simulink model "simulinkCS"  (Simulink 7.4)
settings: Solver=ode45  StartTime=0.0  StopTime=10.0  RelTol=1e-3
(part 1 of 2)
settings Model: Creator=Kubik  LastModifiedBy=Kubik

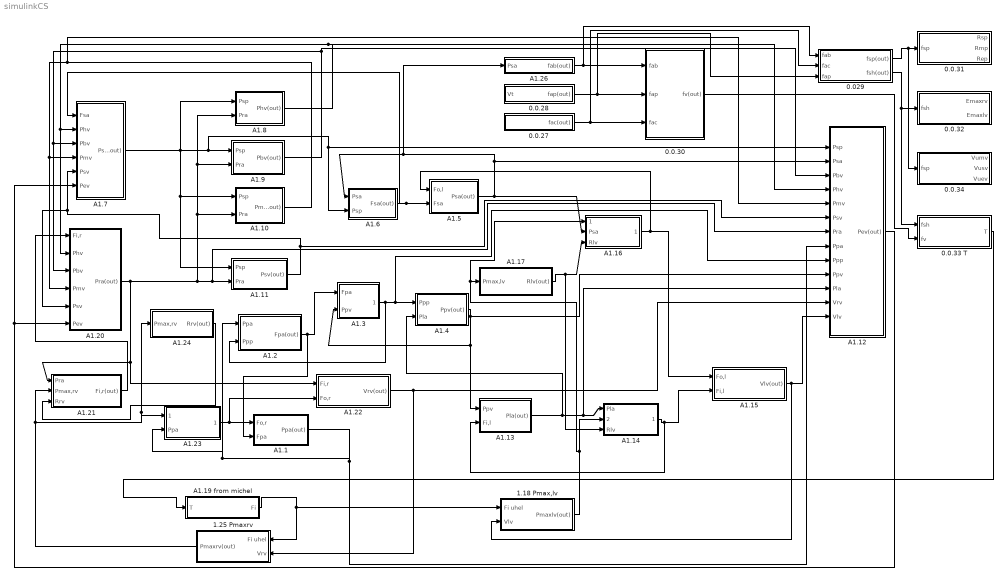
== system simulinkCS ==
  0.0.27 : Subsystem
  0.0.28 : Subsystem
  0.0.30 : Subsystem
  0.0.31 : Subsystem
  0.0.32 : Subsystem
  0.0.33 T : Subsystem
  0.0.34 : Subsystem
  0.029 : Subsystem
  1.18 Pmax,lv : Subsystem
  1.25 Pmaxrv : Subsystem
  A1.1 : Subsystem
  A1.10 : Subsystem
  A1.11 : Subsystem
  A1.12 : Subsystem
  A1.13 : Subsystem
  A1.14 : Subsystem
  A1.15 : Subsystem
  A1.16 : Subsystem
  A1.17 : Subsystem
  A1.19 from michel : Subsystem
  A1.2 : Subsystem
  A1.20 : Subsystem
  A1.21 : Subsystem
  A1.22 : Subsystem
  A1.23 : Subsystem
  A1.24 : Subsystem
  A1.26 : Subsystem
  A1.3 : Subsystem
  A1.4 : Subsystem
  A1.5 : Subsystem
  A1.6 : Subsystem
  A1.7 : Subsystem
  A1.8 : Subsystem
  A1.9 : Subsystem
  wires:
  A1.14/1(Fi,l(out)) -> A1.15/2(Fi,l), A1.13/2(Fi,l)
  A1.16/1(Fo,l(out)) -> A1.15/1(Fo,l), A1.5/1(Fo,l)
  A1.17/1(Rlv(out)) -> A1.16/3(Rlv), A1.14/3(Rlv)
  A1.5/1(Psa(out)) -> A1.16/2(Psa), A1.6/1(Psa), A1.26/1(Psa), A1.12/2(Psa)
  A1.13/1(Pla(out)) -> A1.4/2(Pla), A1.14/1(Pla), A1.12/11(Pla)
  A1.20/1(Pra(out)) -> A1.10/2(Pra), A1.9/2(Pra), A1.8/2(Pra), A1.11/2(Pra), A1.12/7(Pra), A1.21/1(Pra), A1.22/1(Fi,r)
  A1.7/1(Psp(out)) -> A1.8/1(Psp), A1.10/1(Psp), A1.11/1(Psp), A1.9/1(Psp), A1.6/2(Psp), A1.12/1(Psp)
  A1.15/1(Vlv(out)) -> A1.12/13(Vlv), 1.18 Pmax,lv/2(Vlv)
  A1.6/1(Fsa(out)) -> A1.5/2(Fsa), A1.7/1(Fsa)
  A1.21/1(Fi,r(out)) -> A1.20/1(Fi,r)
  A1.23/1(Fo,r(out)) -> A1.1/1(Fo,r), A1.22/2(Fo,r)
  A1.1/1(Ppa(out)) -> A1.23/2(Ppa), A1.2/1(Ppa), A1.12/8(Ppa)
  A1.22/1(Vrv(out)) -> A1.12/12(Vrv), 1.25 Pmaxrv/2(Vrv)
  A1.4/1(Ppv(out)) -> A1.13/1(Ppv), A1.3/2(Ppv), A1.12/10(Ppv)
  A1.3/1(Ppp(out)) -> A1.2/2(Ppp), A1.4/1(Ppp), A1.12/9(Ppp)
  A1.26/1(fab(out)) -> 0.0.30/1(fab), 0.029/1(fab)
  A1.2/1(Fpa(out)) -> A1.3/1(Fpa), A1.1/2(Fpa)
  A1.11/1(Psv(out)) -> A1.7/5(Psv), A1.20/5(Psv), A1.12/6(Psv)
  A1.10/1(Pmv(out)) -> A1.7/4(Pmv), A1.20/4(Pmv), A1.12/5(Pmv)
  A1.9/1(Pbv(out)) -> A1.7/3(Pbv), A1.20/3(Pbv), A1.12/3(Pbv)
  A1.8/1(Phv(out)) -> A1.7/2(Phv), A1.20/2(Phv), A1.12/4(Phv)
  0.0.27/1(fac(out)) -> 0.0.30/3(fac), 0.029/2(fac)
  0.0.28/1(fap(out)) -> 0.0.30/2(fap), 0.029/3(fap)
  A1.12/1(Pev(out)) -> A1.20/6(Pev), A1.7/6(Pev)
  A1.24/1(Rrv(out)) -> A1.21/3(Rrv)
  A1.19 from michel/1(Fi) -> 1.25 Pmaxrv/1(Fi uhel), 1.18 Pmax,lv/1(Fi uhel)
  1.25 Pmaxrv/1(Pmaxrv(out)) -> A1.21/2(Pmax,rv), A1.24/1(Pmax,rv), A1.23/1(Pmax,rv)
  1.18 Pmax,lv/1(Pmaxlv(out)) -> A1.14/2(Pmax,lv), A1.17/1(Pmax,lv), A1.16/1(Pmax,lv)
  0.029/1(fsp(out)) -> 0.0.31/1(fsp), 0.0.34/1(fsp)
  0.029/2(fsh(out)) -> 0.0.32/1(fsh), 0.0.33 T/1(fsh)
  0.0.30/1(fv(out)) -> 0.0.33 T/2(fv)
  0.0.33 T/1(T) -> A1.19 from michel/1(T)

== system simulinkCS/0.0.27 ==
  1 : Constant  OutDataType=fixdt(1, 16)  OutScaling=2^0
  Add : Sum  OutDataType=fixdt(1, 16)  OutScaling=2^-10
  Add1 : Sum  Inputs=+-  OutDataType=fixdt(1, 16)  OutScaling=2^-10
  Add2 : Sum  OutDataType=fixdt(1, 16)  OutScaling=2^-10
  Add4 : Sum  Inputs=-+  OutDataType=fixdt(1, 16)  OutScaling=2^-10
  Divide : Product  Inputs=*/  OutDataType=fixdt(1, 16)  OutScaling=2^-10
  Divide1 : Product  Inputs=*/  OutDataType=fixdt(1, 16)  OutScaling=2^-10
  Divide2 : Product  Inputs=*/  OutDataType=fixdt(1, 16)  OutScaling=2^-10
  Integrator1 : Integrator
  Math Function : Math  OutDataType=fixdt(1, 16)  OutScaling=2^0  SaturateOnIntegerOverflow=on
  Pas,O2 : Constant  Value=35  OutMin=30  OutMax=110  OutDataType=fixdt(1, 16)  OutScaling=2^0
  Pas,O2n : Constant  Value=45  OutDataType=fixdt(1, 16)  OutScaling=2^0
  Product : Product  OutDataType=fixdt(1, 16)  OutScaling=2^0  RndMeth=Zero
  fac,max : Constant  Value=2.52  OutDataType=fixdt(1, 16)  OutScaling=2^0
  fac,min : Constant  Value=47.78  OutDataType=fixdt(1, 16)  OutScaling=2^0
  kac : Constant  Value=29.27  OutDataType=fixdt(1, 16)  OutScaling=2^0
  tau-c : Constant  OutDataType=fixdt(1, 16)  OutScaling=2^0
  fac(out) : Outport  OutDataType=fixdt(1, 16)  OutScaling=2^0
  wires:
  Integrator1/1 -> fac(out)/1, Add4/1
  Add4/1 -> Divide2/1
  Divide2/1 -> Integrator1/1
  tau-c/1 -> Divide2/2
  fac,min/1 -> Product/1
  Math Function/1 -> Product/2, Add2/1
  Add/1 -> Divide/1
  Product/1 -> Add/2
  fac,max/1 -> Add/1
  1/1 -> Add2/2
  Add2/1 -> Divide/2
  Divide/1 -> Add4/2
  Add1/1 -> Divide1/1
  kac/1 -> Divide1/2
  Divide1/1 -> Math Function/1
  Pas,O2n/1 -> Add1/2
  Pas,O2/1 -> Add1/1

== system simulinkCS/0.0.28 ==
  Vt : Inport  OutDataType=fixdt(1, 16)  OutScaling=2^0
  Add4 : Sum  Inputs=-+  OutDataType=fixdt(1, 16)  OutScaling=2^-10
  Divide2 : Product  Inputs=*/  OutDataType=fixdt(1, 16)  OutScaling=2^-10
  Gap : Constant  Value=1000/23291  OutDataType=fixdt(1, 16)  OutScaling=2^0
  Integrator1 : Integrator
  Product : Product  OutDataType=fixdt(1, 16)  OutScaling=2^0  RndMeth=Zero
  tau-c : Constant  OutDataType=fixdt(1, 16)  OutScaling=2^0
  fap(out) : Outport  OutDataType=fixdt(1, 16)  OutScaling=2^0
  wires:
  Integrator1/1 -> fap(out)/1, Add4/1
  Add4/1 -> Divide2/1
  Divide2/1 -> Integrator1/1
  tau-c/1 -> Divide2/2
  Gap/1 -> Product/1
  Product/1 -> Add4/2
  Vt/1 -> Product/2

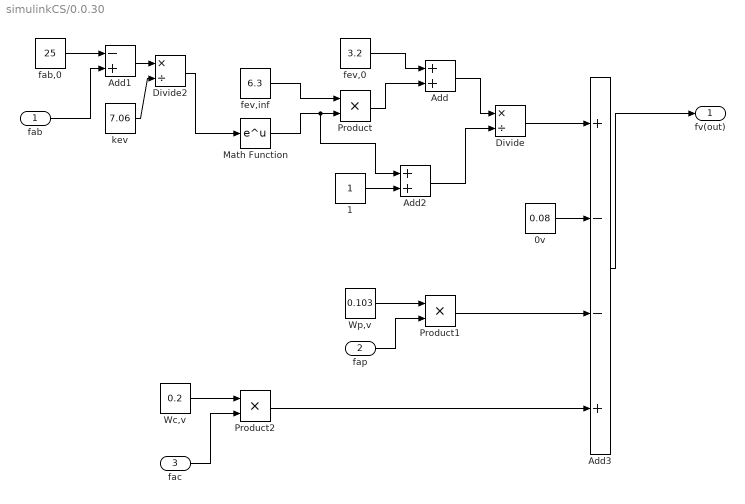
== system simulinkCS/0.0.30 ==
  fab : Inport  OutDataType=fixdt(1, 16)  OutScaling=2^0
  fap : Inport  Port=2  OutDataType=fixdt(1, 16)  OutScaling=2^0
  fac : Inport  Port=3  OutDataType=fixdt(1, 16)  OutScaling=2^0
  0v : Constant  Value=0.08  OutDataType=fixdt(1, 16)  OutScaling=2^0
  1 : Constant  OutDataType=fixdt(1, 16)  OutScaling=2^0
  Add : Sum  OutDataType=fixdt(1, 16)  OutScaling=2^-10
  Add1 : Sum  Inputs=-+  OutDataType=fixdt(1, 16)  OutScaling=2^-10
  Add2 : Sum  OutDataType=fixdt(1, 16)  OutScaling=2^-10
  Add3 : Sum  Inputs=+--+  OutDataType=fixdt(1, 16)  OutScaling=2^-10
  Divide : Product  Inputs=*/  OutDataType=fixdt(1, 16)  OutScaling=2^-10
  Divide2 : Product  Inputs=*/  OutDataType=fixdt(1, 16)  OutScaling=2^-10
  Math Function : Math  OutDataType=fixdt(1, 16)  OutScaling=2^0  SaturateOnIntegerOverflow=on
  Product : Product  OutDataType=fixdt(1, 16)  OutScaling=2^0  RndMeth=Zero
  Product1 : Product  OutDataType=fixdt(1, 16)  OutScaling=2^0  RndMeth=Zero
  Product2 : Product  OutDataType=fixdt(1, 16)  OutScaling=2^0  RndMeth=Zero
  Wc,v : Constant  Value=0.2  OutDataType=fixdt(1, 16)  OutScaling=2^0
  Wp,v : Constant  Value=0.103  OutDataType=fixdt(1, 16)  OutScaling=2^0
  fab,0 : Constant  Value=25  OutDataType=fixdt(1, 16)  OutScaling=2^0
  fev,0 : Constant  Value=3.2  OutDataType=fixdt(1, 16)  OutScaling=2^0
  fev,inf : Constant  Value=6.3  OutDataType=fixdt(1, 16)  OutScaling=2^0
  kev : Constant  Value=7.06  OutDataType=fixdt(1, 16)  OutScaling=2^0
  fv(out) : Outport  OutDataType=fixdt(1, 16)  OutScaling=2^0
  wires:
  fev,inf/1 -> Product/1
  Math Function/1 -> Product/2, Add2/1
  Add/1 -> Divide/1
  Product/1 -> Add/2
  fev,0/1 -> Add/1
  Add1/1 -> Divide2/1
  Divide2/1 -> Math Function/1
  kev/1 -> Divide2/2
  fab,0/1 -> Add1/1
  1/1 -> Add2/2
  Add2/1 -> Divide/2
  fab/1 -> Add1/2
  Divide/1 -> Add3/1
  Add3/1 -> fv(out)/1
  0v/1 -> Add3/2
  Wp,v/1 -> Product1/1
  Wc,v/1 -> Product2/1
  Product1/1 -> Add3/3
  Product2/1 -> Add3/4
  fap/1 -> Product1/2
  fac/1 -> Product2/2

== system simulinkCS/0.0.31 ==
  fsp : Inport  OutDataType=sfix(16)  OutScaling=2^0
  Rep sub : Subsystem
  Rmp sub : Subsystem
  Rsp sub : Subsystem
  Rsp : Outport  OutDataType=sfix(16)  OutScaling=2^0
  Rmp : Outport  Port=2  OutDataType=sfix(16)  OutScaling=2^0
  Rep : Outport  Port=3  OutDataType=sfix(16)  OutScaling=2^0
  wires:
  fsp/1 -> Rsp sub/1(fsp), Rmp sub/1(fsp), Rep sub/1(fsp)
  Rsp sub/1(Rsp) -> Rsp/1
  Rmp sub/1(Rmp) -> Rmp/1
  Rep sub/1(Rep) -> Rep/1

== system simulinkCS/0.0.32 ==
  fsh : Inport  OutDataType=sfix(16)  OutScaling=2^0
  Rmp sub : Subsystem
  Rsp sub : Subsystem
  Emaxrv : Outport  OutDataType=sfix(16)  OutScaling=2^0
  Emaxlv : Outport  Port=2  OutDataType=sfix(16)  OutScaling=2^0
  wires:
  fsh/1 -> Rsp sub/1(fsh), Rmp sub/1(fsh)
  Rsp sub/1(Emaxrv) -> Emaxrv/1
  Rmp sub/1(Emaxlv) -> Emaxlv/1

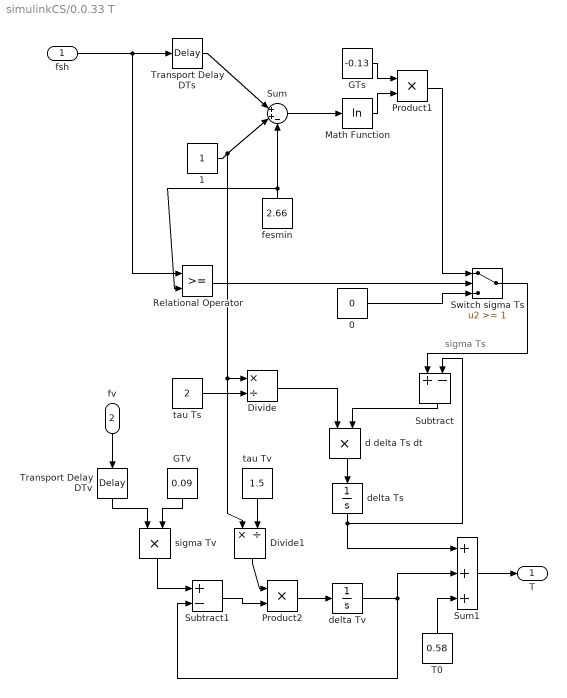
== system simulinkCS/0.0.33 T ==
  note: sigma Ts
  fsh : Inport  OutDataType=sfix(16)  OutScaling=2^0
  fv : Inport  Port=2  OutDataType=sfix(16)  OutScaling=2^0
  0 : Constant  Value=0  OutDataType=sfix(16)  OutScaling=2^0
  1 : Constant  OutDataType=sfix(16)  OutScaling=2^0
  Divide : Product  Inputs=*/  OutDataType=sfix(16)  OutScaling=2^-10
  Divide1 : Product  Inputs=*/  OutDataType=sfix(16)  OutScaling=2^-10
  GTs : Constant  Value=-0.13  OutDataType=sfix(16)  OutScaling=2^0
  GTv : Constant  Value=0.09  OutDataType=sfix(16)  OutScaling=2^0
  Math Function : Math  Operator=log  OutDataType=sfix(16)  OutScaling=2^0  SaturateOnIntegerOverflow=on
  Product1 : Product  OutDataType=sfix(16)  OutScaling=2^0  RndMeth=Zero
  Product2 : Product  OutDataType=sfix(16)  OutScaling=2^0  RndMeth=Zero
  Relational Operator : RelationalOperator  LogicOutDataTypeMode=boolean  OutDataTypeStr=boolean
  Subtract : Sum  Inputs=+-  OutDataType=sfix(16)  OutScaling=2^-10
  Subtract1 : Sum  Inputs=+-  OutDataType=sfix(16)  OutScaling=2^-10
  Sum : Sum  Inputs=|++-  OutDataType=sfix(16)  OutScaling=2^0
  Sum1 : Sum  Inputs=+++  OutDataType=sfix(16)  OutScaling=2^0
  Switch sigma Ts : Switch  Threshold=1
  T0 : Constant  Value=0.58  OutDataType=sfix(16)  OutScaling=2^0
  Transport Delay DTs : TransportDelay  DelayTime=2
  Transport Delay DTv : TransportDelay  DelayTime=0.2
  "d delta Ts dt  " : Product  OutDataType=sfix(16)  OutScaling=2^0  RndMeth=Zero
  delta Ts : Integrator
  delta Tv : Integrator
  fesmin : Constant  Value=2.66  OutDataType=sfix(16)  OutScaling=2^0
  sigma Tv : Product  OutDataType=sfix(16)  OutScaling=2^0  RndMeth=Zero
  tau Ts : Constant  Value=2  OutDataType=sfix(16)  OutScaling=2^0
  tau Tv : Constant  Value=1.5  OutDataType=sfix(16)  OutScaling=2^0
  T : Outport  OutDataType=sfix(16)  OutScaling=2^0
  wires:
  fsh/1 -> Transport Delay DTs/1, Relational Operator/1
  GTs/1 -> Product1/1
  1/1 -> Sum/2, Divide/1, Divide1/1
  fesmin/1 -> Sum/3, Relational Operator/2
  Transport Delay DTs/1 -> Sum/1
  Sum/1 -> Math Function/1
  Math Function/1 -> Product1/2
  Product1/1 -> Switch sigma Ts/1
  Relational Operator/1 -> Switch sigma Ts/2
  0/1 -> Switch sigma Ts/3
  Switch sigma Ts/1 -> Subtract/1
  tau Ts/1 -> Divide/2
  delta Ts/1 -> Subtract/2, Sum1/1
  Subtract/1 -> "d delta Ts dt  "/2
  Divide/1 -> "d delta Ts dt  "/1
  "d delta Ts dt  "/1 -> delta Ts/1
  fv/1 -> Transport Delay DTv/1
  Transport Delay DTv/1 -> sigma Tv/1
  GTv/1 -> sigma Tv/2
  tau Tv/1 -> Divide1/2
  sigma Tv/1 -> Subtract1/1
  delta Tv/1 -> Subtract1/2, Sum1/2
  Product2/1 -> delta Tv/1
  Subtract1/1 -> Product2/2
  Divide1/1 -> Product2/1
  T0/1 -> Sum1/3
  Sum1/1 -> T/1

== system simulinkCS/0.0.34 ==
  fsp : Inport  OutDataType=sfix(16)  OutScaling=2^0
  Vumv sub : Subsystem
  Vumv sub1 : Subsystem
  Vumv sub2 : Subsystem
  Vumv : Outport  OutDataType=sfix(16)  OutScaling=2^0
  Vusv : Outport  Port=2  OutDataType=sfix(16)  OutScaling=2^0
  Vuev : Outport  Port=3  OutDataType=sfix(16)  OutScaling=2^0
  wires:
  fsp/1 -> Vumv sub/1(fsp), Vumv sub1/1(fsp), Vumv sub2/1(fsp)
  Vumv sub/1(Vumv) -> Vumv/1
  Vumv sub1/1(Vusv) -> Vusv/1
  Vumv sub2/1(Vuev) -> Vuev/1

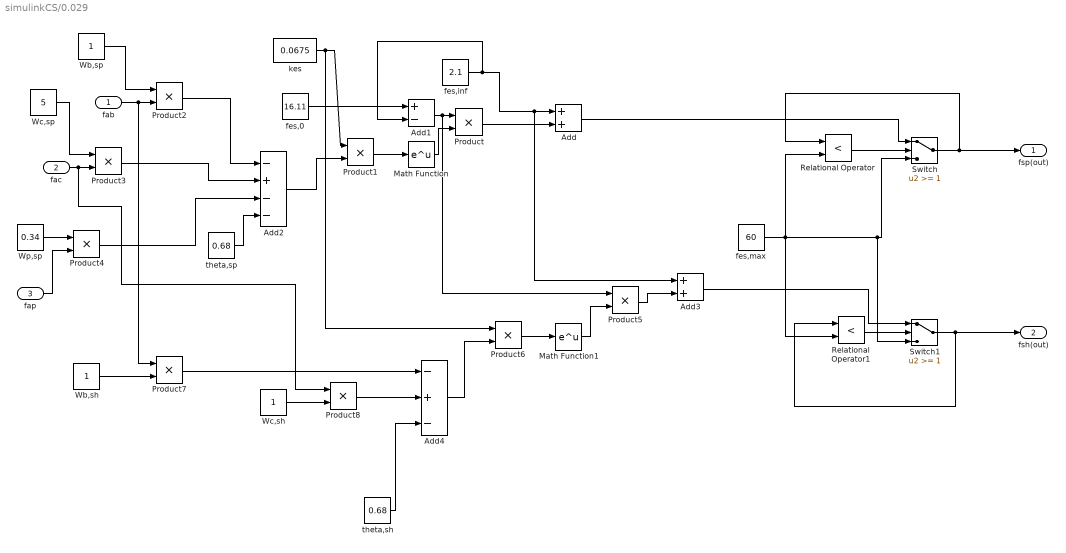
== system simulinkCS/0.029 ==
  fab : Inport  OutDataType=fixdt(1, 16)  OutScaling=2^0
  fac : Inport  Port=2  OutDataType=fixdt(1, 16)  OutScaling=2^0
  fap : Inport  Port=3  OutDataType=fixdt(1, 16)  OutScaling=2^0
  Add : Sum  OutDataType=fixdt(1, 16)  OutScaling=2^-10
  Add1 : Sum  Inputs=+-  OutDataType=fixdt(1, 16)  OutScaling=2^-10
  Add2 : Sum  Inputs=-+--  OutDataType=fixdt(1, 16)  OutScaling=2^-10
  Add3 : Sum  OutDataType=fixdt(1, 16)  OutScaling=2^-10
  Add4 : Sum  Inputs=-+-  OutDataType=fixdt(1, 16)  OutScaling=2^-10
  Math Function : Math  OutDataType=fixdt(1, 16)  OutScaling=2^0  SaturateOnIntegerOverflow=on
  Math Function1 : Math  OutDataType=fixdt(1, 16)  OutScaling=2^0  SaturateOnIntegerOverflow=on
  Product{,1..8} (9 alike) : Product  OutDataType=fixdt(1, 16)  OutScaling=2^0  RndMeth=Zero
  Relational Operator : RelationalOperator  Operator=<  LogicOutDataTypeMode=boolean  LogicDataType=fixdt(0, 8)  OutDataTypeStr=boolean
  Relational Operator1 : RelationalOperator  Operator=<  LogicOutDataTypeMode=boolean  LogicDataType=fixdt(0, 8)  OutDataTypeStr=boolean
  Switch : Switch  Threshold=1  OutDataType=fixdt(1, 16)  OutScaling=2^0
  Switch1 : Switch  Threshold=1  OutDataType=fixdt(1, 16)  OutScaling=2^0
  Wb,sh : Constant  OutDataType=fixdt(1, 16)  OutScaling=2^0
  Wb,sp : Constant  OutDataType=fixdt(1, 16)  OutScaling=2^0
  Wc,sh : Constant  OutDataType=fixdt(1, 16)  OutScaling=2^0
  Wc,sp : Constant  Value=5  OutDataType=fixdt(1, 16)  OutScaling=2^0
  Wp,sp : Constant  Value=0.34  OutDataType=fixdt(1, 16)  OutScaling=2^0
  fes,0 : Constant  Value=16.11  OutDataType=fixdt(1, 16)  OutScaling=2^0
  fes,inf : Constant  Value=2.1  OutDataType=fixdt(1, 16)  OutScaling=2^0
  fes,max : Constant  Value=60  OutDataType=fixdt(1, 16)  OutScaling=2^0
  kes : Constant  Value=0.0675  OutDataType=fixdt(1, 16)  OutScaling=2^0
  theta,sh : Constant  Value=0.68  OutDataType=fixdt(1, 16)  OutScaling=2^0
  theta,sp : Constant  Value=0.68  OutDataType=fixdt(1, 16)  OutScaling=2^0
  fsp(out) : Outport  OutDataType=fixdt(1, 16)  OutScaling=2^0
  fsh(out) : Outport  Port=2  OutDataType=fixdt(1, 16)  OutScaling=2^0
  wires:
  Switch/1 -> fsp(out)/1, Relational Operator/1
  Switch1/1 -> fsh(out)/1, Relational Operator1/1
  fes,max/1 -> Switch1/3, Switch/3, Relational Operator/2, Relational Operator1/2
  Relational Operator1/1 -> Switch1/2
  Relational Operator/1 -> Switch/2
  Add1/1 -> Product/1, Product5/1
  Product/1 -> Add/2
  fes,inf/1 -> Add1/2, Add/1, Add3/1
  Math Function/1 -> Product/2
  Add/1 -> Switch/1
  fes,0/1 -> Add1/1
  Product1/1 -> Math Function/1
  Add2/1 -> Product1/2
  kes/1 -> Product1/1, Product6/1
  Product2/1 -> Add2/1
  fab/1 -> Product2/2, Product7/1
  Product3/1 -> Add2/2
  fac/1 -> Product3/2, Product8/1
  Product4/1 -> Add2/3
  theta,sp/1 -> Add2/4
  Wp,sp/1 -> Product4/1
  Wb,sp/1 -> Product2/1
  Add3/1 -> Switch1/1
  Product5/1 -> Add3/2
  Math Function1/1 -> Product5/2
  Product6/1 -> Math Function1/1
  Add4/1 -> Product6/2
  theta,sh/1 -> Add4/3
  Product7/1 -> Add4/1
  Wb,sh/1 -> Product7/2
  Wc,sp/1 -> Product3/1
  fap/1 -> Product4/2
  Product8/1 -> Add4/2
  Wc,sh/1 -> Product8/2

== system simulinkCS/1.18 Pmax,lv ==
  Fi uhel : Inport  OutDataType=sfix(16)  OutScaling=2^0
  Vlv : Inport  Port=2  OutDataType=sfix(16)  OutScaling=2^0
  1 : Constant  OutDataType=sfix(16)  OutScaling=2^0
  Add : Sum  OutDataType=sfix(16)  OutScaling=2^-10
  Emax : Constant  Value=2.95  OutDataType=sfix(16)  OutScaling=2^0
  Math Function : Math  OutDataType=sfix(16)  OutScaling=2^0  SaturateOnIntegerOverflow=on
  Polv : Constant  Value=1.5  OutDataType=sfix(16)  OutScaling=2^0
  Product : Product  Inputs=3  OutDataType=sfix(16)  OutScaling=2^0  RndMeth=Zero
  Product1 : Product  OutDataType=sfix(16)  OutScaling=2^0  RndMeth=Zero
  Product2 : Product  Inputs=3  OutDataType=sfix(16)  OutScaling=2^0  RndMeth=Zero
  Subtract : Sum  Inputs=+-  OutDataType=sfix(16)  OutScaling=2^-10
  Subtract1 : Sum  Inputs=+-  OutDataType=sfix(16)  OutScaling=2^-10
  Subtract2 : Sum  Inputs=+-  OutDataType=sfix(16)  OutScaling=2^-10
  Vulv : Constant  Value=16.77  OutDataType=sfix(16)  OutScaling=2^0
  kElv : Constant  Value=0.014  OutDataType=sfix(16)  OutScaling=2^0
  Pmaxlv(out) : Outport  OutDataType=sfix(16)  OutScaling=2^0
  wires:
  Vlv/1 -> Subtract/1, Product1/1
  Vulv/1 -> Subtract/2
  Subtract/1 -> Product/3
  Emax/1 -> Product/2
  Fi uhel/1 -> Product/1, Subtract2/2
  kElv/1 -> Product1/2
  Product1/1 -> Math Function/1
  Math Function/1 -> Subtract1/1
  1/1 -> Subtract1/2, Subtract2/1
  Polv/1 -> Product2/1
  Subtract1/1 -> Product2/2
  Subtract2/1 -> Product2/3
  Product/1 -> Add/1
  Product2/1 -> Add/2
  Add/1 -> Pmaxlv(out)/1

== system simulinkCS/1.25 Pmaxrv ==
  Fi uhel : Inport  OutDataType=sfix(16)  OutScaling=2^0
  Vrv : Inport  Port=2  OutDataType=sfix(16)  OutScaling=2^0
  1 : Constant  OutDataType=sfix(16)  OutScaling=2^0
  Add : Sum  OutDataType=sfix(16)  OutScaling=2^-10
  Emaxrv : Constant  Value=1.75  OutDataType=sfix(16)  OutScaling=2^0
  Math Function : Math  OutDataType=sfix(16)  OutScaling=2^0  SaturateOnIntegerOverflow=on
  Polv : Constant  Value=1.5  OutDataType=sfix(16)  OutScaling=2^0
  Product : Product  Inputs=3  OutDataType=sfix(16)  OutScaling=2^0  RndMeth=Zero
  Product1 : Product  OutDataType=sfix(16)  OutScaling=2^0  RndMeth=Zero
  Product2 : Product  Inputs=3  OutDataType=sfix(16)  OutScaling=2^0  RndMeth=Zero
  Subtract : Sum  Inputs=+-  OutDataType=sfix(16)  OutScaling=2^-10
  Subtract1 : Sum  Inputs=+-  OutDataType=sfix(16)  OutScaling=2^-10
  Subtract2 : Sum  Inputs=+-  OutDataType=sfix(16)  OutScaling=2^-10
  Vurv : Constant  Value=40.8  OutDataType=sfix(16)  OutScaling=2^0
  kErv : Constant  Value=0.011  OutDataType=sfix(16)  OutScaling=2^0
  Pmaxrv(out) : Outport  OutDataType=sfix(16)  OutScaling=2^0
  wires:
  Vrv/1 -> Subtract/1, Product1/1
  Vurv/1 -> Subtract/2
  Subtract/1 -> Product/3
  Emaxrv/1 -> Product/2
  Fi uhel/1 -> Product/1, Subtract2/2
  kErv/1 -> Product1/2
  Product1/1 -> Math Function/1
  Math Function/1 -> Subtract1/1
  1/1 -> Subtract1/2, Subtract2/1
  Polv/1 -> Product2/1
  Subtract1/1 -> Product2/2
  Subtract2/1 -> Product2/3
  Product/1 -> Add/1
  Product2/1 -> Add/2
  Add/1 -> Pmaxrv(out)/1

== system simulinkCS/A1.1 ==
  Fo,r : Inport  OutDataType=fixdt(1, 16)  OutScaling=2^0
  Fpa : Inport  Port=2  OutDataType=fixdt(1, 16)  OutScaling=2^0
  Cpa : Constant  Value=0.76  OutDataType=fixdt(1, 16)  OutScaling=2^0
  Divide : Product  Inputs=*/  OutDataType=fixdt(1, 16)  OutScaling=2^-10
  Integrator : Integrator
  Subtract : Sum  Inputs=+-  OutDataType=fixdt(1, 16)  OutScaling=2^-10
  Ppa(out) : Outport  OutDataType=fixdt(1, 16)  OutScaling=2^0
  wires:
  Cpa/1 -> Divide/2
  Fo,r/1 -> Subtract/1
  Fpa/1 -> Subtract/2
  Subtract/1 -> Divide/1
  Divide/1 -> Integrator/1
  Integrator/1 -> Ppa(out)/1

== system simulinkCS/A1.10 ==
  Psp : Inport  OutDataType=fixdt(1, 16)  OutScaling=2^0
  Pra : Inport  Port=2  OutDataType=fixdt(1, 16)  OutScaling=2^0
  Cmv : Constant  Value=15.71  OutDataType=fixdt(1, 16)  OutScaling=2^0
  Derivative : Derivative
  Divide : Product  Inputs=*/  OutDataType=fixdt(1, 16)  OutScaling=2^-10
  Divide1 : Product  Inputs=*/  OutDataType=fixdt(1, 16)  OutScaling=2^-10
  Divide2 : Product  Inputs=/*  OutDataType=fixdt(1, 16)  OutScaling=2^-10
  Integrator : Integrator
  Rmp : Constant  Value=4.48  OutDataType=fixdt(1, 16)  OutScaling=2^0
  Rmv : Constant  Value=0.05  OutDataType=fixdt(1, 16)  OutScaling=2^0
  Subtract : Sum  Inputs=+--  OutDataType=fixdt(1, 16)  OutScaling=2^-10
  Sum : Sum  Inputs=|+-  OutDataType=fixdt(1, 16)  OutScaling=2^0
  Sum1 : Sum  Inputs=|-+  OutDataType=fixdt(1, 16)  OutScaling=2^0
  Vu,mv : Constant  Value=432.14  OutDataType=fixdt(1, 16)  OutScaling=2^0
  Pmv(out) : Outport  OutDataType=fixdt(1, 16)  OutScaling=2^0
  wires:
  Integrator/1 -> Pmv(out)/1, Sum/2, Sum1/2
  Psp/1 -> Sum/1
  Sum/1 -> Divide1/1
  Rmp/1 -> Divide1/2
  Pra/1 -> Sum1/1
  Sum1/1 -> Divide2/2
  Rmv/1 -> Divide2/1
  Divide1/1 -> Subtract/1
  Divide2/1 -> Subtract/2
  Cmv/1 -> Divide/2
  Divide/1 -> Integrator/1
  Vu,mv/1 -> Derivative/1
  Derivative/1 -> Subtract/3
  Subtract/1 -> Divide/1

== system simulinkCS/A1.11 ==
  Psp : Inport  OutDataType=fixdt(1, 16)  OutScaling=2^0
  Pra : Inport  Port=2  OutDataType=fixdt(1, 16)  OutScaling=2^0
  Csv : Constant  Value=61.11  OutDataType=fixdt(1, 16)  OutScaling=2^0
  Derivative : Derivative
  Divide : Product  Inputs=*/  OutDataType=fixdt(1, 16)  OutScaling=2^-10
  Divide1 : Product  Inputs=*/  OutDataType=fixdt(1, 16)  OutScaling=2^-10
  Divide2 : Product  Inputs=/*  OutDataType=fixdt(1, 16)  OutScaling=2^-10
  Integrator : Integrator
  Rsp : Constant  Value=3.307  OutDataType=fixdt(1, 16)  OutScaling=2^0
  Rsv : Constant  Value=0.038  OutDataType=fixdt(1, 16)  OutScaling=2^0
  Subtract : Sum  Inputs=+--  OutDataType=fixdt(1, 16)  OutScaling=2^-10
  Sum : Sum  Inputs=|+-  OutDataType=fixdt(1, 16)  OutScaling=2^0
  Sum1 : Sum  Inputs=|-+  OutDataType=fixdt(1, 16)  OutScaling=2^0
  Vu,sv : Constant  Value=1.121  OutDataType=fixdt(1, 16)  OutScaling=2^0
  Psv(out) : Outport  OutDataType=fixdt(1, 16)  OutScaling=2^0
  wires:
  Integrator/1 -> Psv(out)/1, Sum/2, Sum1/2
  Psp/1 -> Sum/1
  Sum/1 -> Divide1/1
  Rsp/1 -> Divide1/2
  Pra/1 -> Sum1/1
  Sum1/1 -> Divide2/2
  Rsv/1 -> Divide2/1
  Divide1/1 -> Subtract/1
  Divide2/1 -> Subtract/2
  Subtract/1 -> Divide/1
  Csv/1 -> Divide/2
  Divide/1 -> Integrator/1
  Vu,sv/1 -> Derivative/1
  Derivative/1 -> Subtract/3

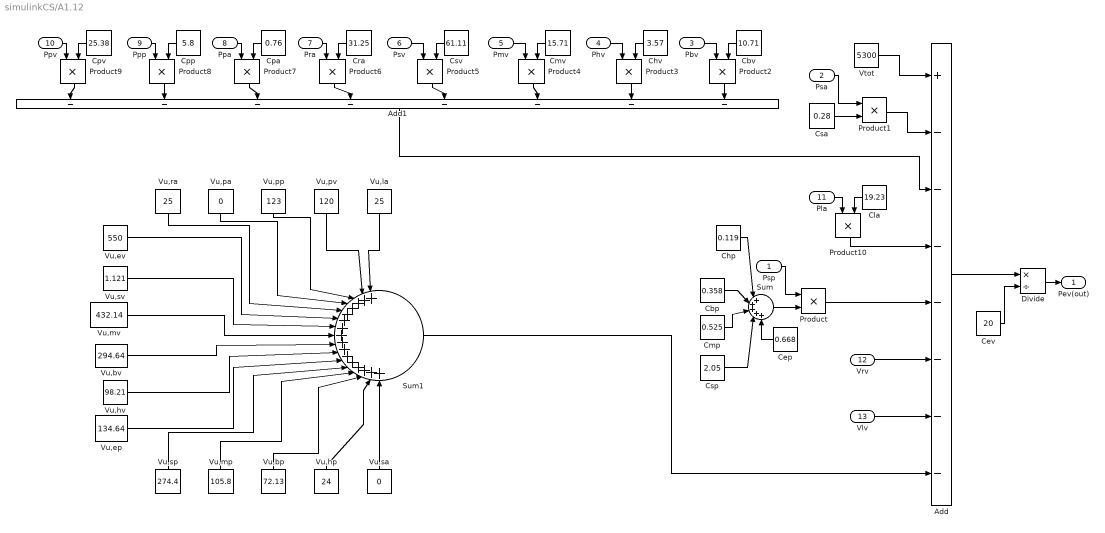
== system simulinkCS/A1.12 ==
  Psp : Inport  OutDataType=fixdt(1, 16)  OutScaling=2^0
  Psa : Inport  Port=2  OutDataType=fixdt(1, 16)  OutScaling=2^0
  Pbv : Inport  Port=3  OutDataType=fixdt(1, 16)  OutScaling=2^0
  Phv : Inport  Port=4  OutDataType=fixdt(1, 16)  OutScaling=2^0
  Pmv : Inport  Port=5  OutDataType=fixdt(1, 16)  OutScaling=2^0
  Psv : Inport  Port=6  OutDataType=fixdt(1, 16)  OutScaling=2^0
  Pra : Inport  Port=7  OutDataType=fixdt(1, 16)  OutScaling=2^0
  Ppa : Inport  Port=8  OutDataType=fixdt(1, 16)  OutScaling=2^0
  Ppp : Inport  Port=9  OutDataType=fixdt(1, 16)  OutScaling=2^0
  Ppv : Inport  Port=10  OutDataType=fixdt(1, 16)  OutScaling=2^0
  Pla : Inport  Port=11  OutDataType=fixdt(1, 16)  OutScaling=2^0
  Vrv : Inport  Port=12  OutDataType=fixdt(1, 16)  OutScaling=2^0
  Vlv : Inport  Port=13  OutDataType=fixdt(1, 16)  OutScaling=2^0
  Add : Sum  Inputs=+-------  OutDataType=fixdt(1, 16)  OutScaling=2^-10
  Add1 : Sum  Inputs=--------  OutDataType=fixdt(1, 16)  OutScaling=2^-10
  Cbp : Constant  Value=0.358  OutDataType=fixdt(1, 16)  OutScaling=2^0
  Cbv : Constant  Value=10.71  OutDataType=fixdt(1, 16)  OutScaling=2^0
  Cep : Constant  Value=0.668  OutDataType=fixdt(1, 16)  OutScaling=2^0
  Cev : Constant  Value=20  OutDataType=fixdt(1, 16)  OutScaling=2^0
  Chp : Constant  Value=0.119  OutDataType=fixdt(1, 16)  OutScaling=2^0
  Chv : Constant  Value=3.57  OutDataType=fixdt(1, 16)  OutScaling=2^0
  Cla : Constant  Value=19.23  OutDataType=fixdt(1, 16)  OutScaling=2^0
  Cmp : Constant  Value=0.525  OutDataType=fixdt(1, 16)  OutScaling=2^0
  Cmv : Constant  Value=15.71  OutDataType=fixdt(1, 16)  OutScaling=2^0
  Cpa : Constant  Value=0.76  OutDataType=fixdt(1, 16)  OutScaling=2^0
  Cpp : Constant  Value=5.8  OutDataType=fixdt(1, 16)  OutScaling=2^0
  Cpv : Constant  Value=25.38  OutDataType=fixdt(1, 16)  OutScaling=2^0
  Cra : Constant  Value=31.25  OutDataType=fixdt(1, 16)  OutScaling=2^0
  Csa : Constant  Value=0.28  OutDataType=fixdt(1, 16)  OutScaling=2^0
  Csp : Constant  Value=2.05  OutDataType=fixdt(1, 16)  OutScaling=2^0
  Csv : Constant  Value=61.11  OutDataType=fixdt(1, 16)  OutScaling=2^0
  Divide : Product  Inputs=*/  OutDataType=fixdt(1, 16)  OutScaling=2^-10
  Product{,1..10} (11 alike) : Product  OutDataType=fixdt(1, 16)  OutScaling=2^0  RndMeth=Zero
  Sum : Sum  Inputs=|+++++  OutDataType=fixdt(1, 16)  OutScaling=2^0
  Sum1 : Sum  Inputs=|++++++++++++++++  OutDataType=fixdt(1, 16)  OutScaling=2^0
  Vtot : Constant  Value=5300  OutDataType=fixdt(1, 16)  OutScaling=2^0
  Vu,bp : Constant  Value=72.13  OutDataType=fixdt(1, 16)  OutScaling=2^0
  Vu,bv : Constant  Value=294.64  OutDataType=fixdt(1, 16)  OutScaling=2^0
  Vu,ep : Constant  Value=134.64  OutDataType=fixdt(1, 16)  OutScaling=2^0
  Vu,ev : Constant  Value=550  OutDataType=fixdt(1, 16)  OutScaling=2^0
  Vu,hp : Constant  Value=24  OutDataType=fixdt(1, 16)  OutScaling=2^0
  Vu,hv : Constant  Value=98.21  OutDataType=fixdt(1, 16)  OutScaling=2^0
  Vu,la : Constant  Value=25  OutDataType=fixdt(1, 16)  OutScaling=2^0
  Vu,mp : Constant  Value=105.8  OutDataType=fixdt(1, 16)  OutScaling=2^0
  Vu,mv : Constant  Value=432.14  OutDataType=fixdt(1, 16)  OutScaling=2^0
  Vu,pa : Constant  Value=0  OutDataType=fixdt(1, 16)  OutScaling=2^0
  Vu,pp : Constant  Value=123  OutDataType=fixdt(1, 16)  OutScaling=2^0
  Vu,pv : Constant  Value=120  OutDataType=fixdt(1, 16)  OutScaling=2^0
  Vu,ra : Constant  Value=25  OutDataType=fixdt(1, 16)  OutScaling=2^0
  Vu,sa : Constant  Value=0  OutDataType=fixdt(1, 16)  OutScaling=2^0
  Vu,sp : Constant  Value=274.4  OutDataType=fixdt(1, 16)  OutScaling=2^0
  Vu,sv : Constant  Value=1.121  OutDataType=fixdt(1, 16)  OutScaling=2^0
  Pev(out) : Outport  OutDataType=fixdt(1, 16)  OutScaling=2^0
  wires:
  Chp/1 -> Sum/1
  Cbp/1 -> Sum/2
  Cmp/1 -> Sum/3
  Cep/1 -> Sum/5
  Csp/1 -> Sum/4
  Psp/1 -> Product/1
  Sum/1 -> Product/2
  Divide/1 -> Pev(out)/1
  Cev/1 -> Divide/2
  Add/1 -> Divide/1
  Product1/1 -> Add/2
  Csa/1 -> Product1/2
  Psa/1 -> Product1/1
  Pbv/1 -> Product2/1
  Cbv/1 -> Product2/2
  Phv/1 -> Product3/1
  Chv/1 -> Product3/2
  Pmv/1 -> Product4/1
  Cmv/1 -> Product4/2
  Psv/1 -> Product5/1
  Csv/1 -> Product5/2
  Pra/1 -> Product6/1
  Cra/1 -> Product6/2
  Ppa/1 -> Product7/1
  Cpa/1 -> Product7/2
  Ppp/1 -> Product8/1
  Cpp/1 -> Product8/2
  Ppv/1 -> Product9/1
  Cpv/1 -> Product9/2
  Pla/1 -> Product10/1
  Cla/1 -> Product10/2
  Product9/1 -> Add1/1
  Product8/1 -> Add1/2
  Product7/1 -> Add1/3
  Product6/1 -> Add1/4
  Product5/1 -> Add1/5
  Product4/1 -> Add1/6
  Product3/1 -> Add1/7
  Product2/1 -> Add1/8
  Product10/1 -> Add/4
  Add1/1 -> Add/3
  Product/1 -> Add/5
  Vrv/1 -> Add/6
  Vtot/1 -> Add/1
  Sum1/1 -> Add/8
  Vu,la/1 -> Sum1/1
  Vu,pv/1 -> Sum1/2
  Vu,pp/1 -> Sum1/3
  Vu,pa/1 -> Sum1/4
  Vu,ra/1 -> Sum1/5
  Vu,ev/1 -> Sum1/6
  Vu,sv/1 -> Sum1/7
  Vu,mv/1 -> Sum1/8
  Vu,bv/1 -> Sum1/9
  Vu,hv/1 -> Sum1/10
  Vu,ep/1 -> Sum1/11
  Vu,sp/1 -> Sum1/12
  Vu,mp/1 -> Sum1/13
  Vu,sa/1 -> Sum1/16
  Vu,bp/1 -> Sum1/14
  Vu,hp/1 -> Sum1/15
  Vlv/1 -> Add/7

== system simulinkCS/A1.13 ==
  Ppv : Inport  OutDataType=fixdt(1, 16)  OutScaling=2^0
  Fi,l : Inport  Port=2  OutDataType=fixdt(1, 16)  OutScaling=2^0
  Cla : Constant  Value=19.23  OutDataType=fixdt(1, 16)  OutScaling=2^0
  Divide : Product  Inputs=*/  OutDataType=fixdt(1, 16)  OutScaling=2^-10
  Divide1 : Product  Inputs=*/  OutDataType=fixdt(1, 16)  OutScaling=2^-10
  Integrator : Integrator
  Rpv : Constant  Value=0.0056  OutDataType=fixdt(1, 16)  OutScaling=2^0
  Subtract : Sum  Inputs=+-  OutDataType=fixdt(1, 16)  OutScaling=2^-10
  Sum : Sum  Inputs=|+-  OutDataType=fixdt(1, 16)  OutScaling=2^0
  Pla(out) : Outport  OutDataType=fixdt(1, 16)  OutScaling=2^0
  wires:
  Integrator/1 -> Pla(out)/1, Sum/2
  Ppv/1 -> Sum/1
  Sum/1 -> Divide1/1
  Rpv/1 -> Divide1/2
  Divide/1 -> Integrator/1
  Cla/1 -> Divide/2
  Subtract/1 -> Divide/1
  Divide1/1 -> Subtract/1
  Fi,l/1 -> Subtract/2

== system simulinkCS/A1.14 ==
  Pla : Inport  OutDataType=fixdt(1, 16)  OutScaling=2^0
  Pmax,lv : Inport  Port=2  OutDataType=fixdt(1, 16)  OutScaling=2^0
  Rlv : Inport  Port=3  OutDataType=fixdt(1, 16)  OutScaling=2^0
  Constant : Constant  Value=0  OutDataType=fixdt(1, 16)  OutScaling=2^0
  Divide : Product  Inputs=*/  OutDataType=fixdt(1, 16)  OutScaling=2^-10
  Fo,l : Constant  Value=1.5  OutDataType=fixdt(1, 16)  OutScaling=2^0
  Plv : Sum  Inputs=+-  OutDataType=fixdt(1, 16)  OutScaling=2^-10
  Product : Product  OutDataType=fixdt(1, 16)  OutScaling=2^0  RndMeth=Zero
  Relational Operator : RelationalOperator  Operator=<=  LogicOutDataTypeMode=boolean  LogicDataType=fixdt(0, 8)  OutDataTypeStr=boolean
  Rla : Constant  Value=0.0025  OutDataType=fixdt(1, 16)  OutScaling=2^0
  Subtract : Sum  Inputs=+-  OutDataType=fixdt(1, 16)  OutScaling=2^-10
  Switch : Switch  OutDataType=fixdt(1, 16)  OutScaling=2^0
  Fi,l(out) : Outport  OutDataType=fixdt(1, 16)  OutScaling=2^0
  wires:
  Switch/1 -> Fi,l(out)/1
  Constant/1 -> Switch/1
  Divide/1 -> Switch/3
  Pla/1 -> Subtract/1, Relational Operator/1
  Rla/1 -> Divide/2
  Subtract/1 -> Divide/1
  Relational Operator/1 -> Switch/2
  Plv/1 -> Subtract/2
  Pmax,lv/1 -> Plv/1
  Product/1 -> Plv/2
  Rlv/1 -> Product/1
  Fo,l/1 -> Product/2

== system simulinkCS/A1.15 ==
  Fo,l : Inport  OutDataType=fixdt(1, 16)  OutScaling=2^0
  Fi,l : Inport  Port=2  OutDataType=fixdt(1, 16)  OutScaling=2^0
  Integrator : Integrator
  Subtract : Sum  Inputs=+-  OutDataType=fixdt(1, 16)  OutScaling=2^-10
  Vlv(out) : Outport  OutDataType=fixdt(1, 16)  OutScaling=2^0
  wires:
  Integrator/1 -> Vlv(out)/1
  Fi,l/1 -> Subtract/2
  Subtract/1 -> Integrator/1
  Fo,l/1 -> Subtract/1

== system simulinkCS/A1.16 ==
  Pmax,lv : Inport  OutDataType=fixdt(1, 16)  OutScaling=2^0
  Psa : Inport  Port=2  OutDataType=fixdt(1, 16)  OutScaling=2^0
  Rlv : Inport  Port=3  OutDataType=fixdt(1, 16)  OutScaling=2^0
  Constant : Constant  Value=0  OutDataType=fixdt(1, 16)  OutScaling=2^0
  Divide : Product  Inputs=*/  OutDataType=fixdt(1, 16)  OutScaling=2^-10
  Relational Operator : RelationalOperator  Operator=<=  LogicOutDataTypeMode=boolean  LogicDataType=fixdt(0, 8)  OutDataTypeStr=boolean
  Subtract : Sum  Inputs=+-  OutDataType=fixdt(1, 16)  OutScaling=2^-10
  Switch : Switch  Threshold=1  OutDataType=fixdt(1, 16)  OutScaling=2^0
  Fo,l(out) : Outport  OutDataType=fixdt(1, 16)  OutScaling=2^0
  wires:
  Switch/1 -> Fo,l(out)/1
  Constant/1 -> Switch/1
  Divide/1 -> Switch/3
  Pmax,lv/1 -> Subtract/1, Relational Operator/1
  Psa/1 -> Subtract/2, Relational Operator/2
  Subtract/1 -> Divide/1
  Rlv/1 -> Divide/2
  Relational Operator/1 -> Switch/2

== system simulinkCS/A1.17 ==
  Pmax,lv : Inport  OutDataType=fixdt(1, 16)  OutScaling=2^0
  Product : Product  OutDataType=fixdt(1, 16)  OutScaling=2^0  RndMeth=Zero
  kR,lv : Constant  Value=0.000375  OutDataType=fixdt(1, 16)  OutScaling=2^0
  Rlv(out) : Outport  OutDataType=fixdt(1, 16)  OutScaling=2^0
  wires:
  Product/1 -> Rlv(out)/1
  Pmax,lv/1 -> Product/2
  kR,lv/1 -> Product/1

== system simulinkCS/A1.19 from michel ==
  T : Inport  OutDataType=sfix(16)  OutScaling=2^0
  Add : Sum  Inputs=-+  OutDataType=sfix(16)  OutScaling=2^-10
  Add1 : Sum  Inputs=+-  OutDataType=sfix(16)  OutScaling=2^-10
  Divide : Product  Inputs=/**  OutDataType=sfix(16)  OutScaling=2^-10
  Embedded MATLAB Function : Stateflow chart
  Fcn : Fcn  Expr=u^2
  Fcn1 : Fcn  Expr=u^2.2
  Fcn2 : Fcn  Expr=(2^2.2)*(2.2^2)*(((u-0)/(2+2.2))^(2+2.2))
  Logical Operator : Logic  AllPortsSameDT=off  OutDataTypeMode=boolean  OutDataTypeStr=boolean
  Product : Product  OutDataType=sfix(16)  OutScaling=2^0  RndMeth=Zero
  Relational Operator : RelationalOperator  LogicOutDataTypeMode=boolean  OutDataTypeStr=boolean
  Relational Operator1 : RelationalOperator  Operator=<=  LogicOutDataTypeMode=boolean  OutDataTypeStr=boolean
  alpha : Constant  Value=0  OutDataType=sfix(16)  OutScaling=2^0
  beta(H) : Subsystem
  m : Constant  Value=2.2  OutDataType=sfix(16)  OutScaling=2^0
  n : Constant  Value=2  OutDataType=sfix(16)  OutScaling=2^0
  t : Clock
      settings: Decimation=10
  Fi : Outport  OutDataType=sfix(16)  OutScaling=2^0
  wires:
  alpha/1 -> Add/1, Relational Operator/2, beta(H)/2(alpha)
  Relational Operator/1 -> Logical Operator/1
  beta(H)/1(Out1) -> Relational Operator1/2, Add1/1, Fcn2/1
  Relational Operator1/1 -> Logical Operator/2
  Add/1 -> Fcn/1
  Add1/1 -> Fcn1/1
  Fcn1/1 -> Product/1
  Fcn/1 -> Product/2
  Product/1 -> Divide/2
  Fcn2/1 -> Divide/1
  Logical Operator/1 -> Divide/3
  T/1 -> beta(H)/1(H), Embedded MATLAB Function/2(Hmin)
  n/1 -> beta(H)/3(n)
  m/1 -> beta(H)/4(m)
  Divide/1 -> Fi/1
  Embedded MATLAB Function/1(y) -> Add1/2, Add/2, Relational Operator/1, Relational Operator1/1
  t/1 -> Embedded MATLAB Function/1(t)

== system simulinkCS/A1.2 ==
  Ppa : Inport  OutDataType=fixdt(1, 16)  OutScaling=2^0
  Ppp : Inport  Port=2  OutDataType=fixdt(1, 16)  OutScaling=2^0
  Divide : Product  Inputs=*/  OutDataType=fixdt(1, 16)  OutScaling=2^-10
  Integrator : Integrator
  Lpa : Constant  Value=1.8*10^(-4)  OutDataType=fixdt(1, 16)  OutScaling=2^0
  Product : Product  OutDataType=fixdt(1, 16)  OutScaling=2^0  RndMeth=Zero
  Rpa : Constant  Value=0.023  OutDataType=fixdt(1, 16)  OutScaling=2^0
  Sum : Sum  Inputs=|+--  OutDataType=fixdt(1, 16)  OutScaling=2^0
  Fpa(out) : Outport  OutDataType=fixdt(1, 16)  OutScaling=2^0
  wires:
  Ppa/1 -> Sum/1
  Ppp/1 -> Sum/2
  Product/1 -> Sum/3
  Rpa/1 -> Product/1
  Integrator/1 -> Fpa(out)/1, Product/2
  Sum/1 -> Divide/1
  Divide/1 -> Integrator/1
  Lpa/1 -> Divide/2

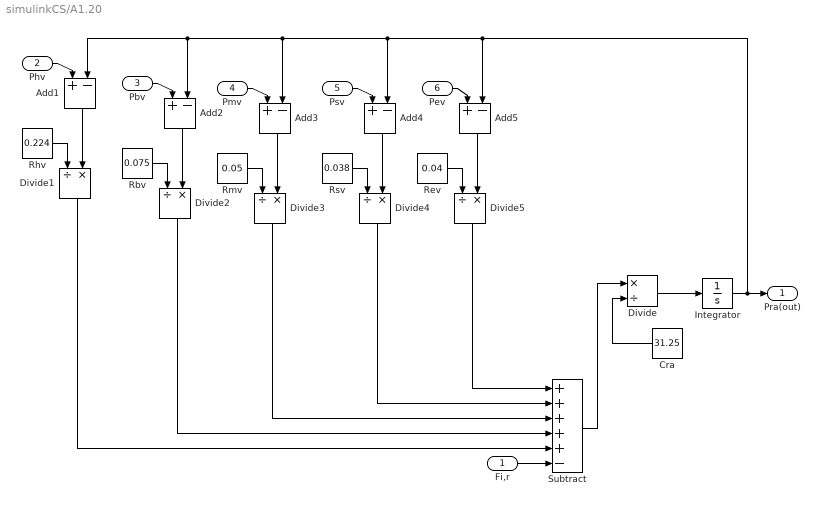
== system simulinkCS/A1.20 ==
  Fi,r : Inport  OutDataType=fixdt(1, 16)  OutScaling=2^0
  Phv : Inport  Port=2  OutDataType=fixdt(1, 16)  OutScaling=2^0
  Pbv : Inport  Port=3  OutDataType=fixdt(1, 16)  OutScaling=2^0
  Pmv : Inport  Port=4  OutDataType=fixdt(1, 16)  OutScaling=2^0
  Psv : Inport  Port=5  OutDataType=fixdt(1, 16)  OutScaling=2^0
  Pev : Inport  Port=6  OutDataType=fixdt(1, 16)  OutScaling=2^0
  Add{1..5} (5 alike) : Sum  Inputs=+-  OutDataType=fixdt(1, 16)  OutScaling=2^-10
  Cra : Constant  Value=31.25  OutDataType=fixdt(1, 16)  OutScaling=2^0
  Divide : Product  Inputs=*/  OutDataType=fixdt(1, 16)  OutScaling=2^-10
  Divide{1..5} (5 alike) : Product  Inputs=/*  OutDataType=fixdt(1, 16)  OutScaling=2^-10
  Integrator : Integrator
  Rbv : Constant  Value=0.075  OutDataType=fixdt(1, 16)  OutScaling=2^0
  Rev : Constant  Value=0.04  OutDataType=fixdt(1, 16)  OutScaling=2^0
  Rhv : Constant  Value=0.224  OutDataType=fixdt(1, 16)  OutScaling=2^0
  Rmv : Constant  Value=0.05  OutDataType=fixdt(1, 16)  OutScaling=2^0
  Rsv : Constant  Value=0.038  OutDataType=fixdt(1, 16)  OutScaling=2^0
  Subtract : Sum  Inputs=+++++-  OutDataType=fixdt(1, 16)  OutScaling=2^-10
  Pra(out) : Outport  OutDataType=fixdt(1, 16)  OutScaling=2^0
  wires:
  Integrator/1 -> Pra(out)/1, Add1/2, Add2/2, Add3/2, Add4/2, Add5/2
  Divide/1 -> Integrator/1
  Cra/1 -> Divide/2
  Subtract/1 -> Divide/1
  Phv/1 -> Add1/1
  Add1/1 -> Divide1/2
  Rhv/1 -> Divide1/1
  Add2/1 -> Divide2/2
  Rbv/1 -> Divide2/1
  Add3/1 -> Divide3/2
  Rmv/1 -> Divide3/1
  Add4/1 -> Divide4/2
  Rsv/1 -> Divide4/1
  Pbv/1 -> Add2/1
  Pmv/1 -> Add3/1
  Psv/1 -> Add4/1
  Add5/1 -> Divide5/2
  Rev/1 -> Divide5/1
  Pev/1 -> Add5/1
  Fi,r/1 -> Subtract/6
  Divide5/1 -> Subtract/1
  Divide4/1 -> Subtract/2
  Divide3/1 -> Subtract/3
  Divide2/1 -> Subtract/4
  Divide1/1 -> Subtract/5

== system simulinkCS/A1.21 ==
  Pra : Inport  OutDataType=fixdt(1, 16)  OutScaling=2^0
  Pmax,rv : Inport  Port=2  OutDataType=fixdt(1, 16)  OutScaling=2^0
  Rrv : Inport  Port=3  OutDataType=fixdt(1, 16)  OutScaling=2^0
  Constant : Constant  Value=0  OutDataType=fixdt(1, 16)  OutScaling=2^0
  Divide : Product  Inputs=*/  OutDataType=fixdt(1, 16)  OutScaling=2^-10
  Fo,r : Constant  Value=1.5  OutDataType=fixdt(1, 16)  OutScaling=2^0
  Product : Product  OutDataType=fixdt(1, 16)  OutScaling=2^0  RndMeth=Zero
  Prv : Sum  Inputs=+-  OutDataType=fixdt(1, 16)  OutScaling=2^-10
  Relational Operator : RelationalOperator  Operator=<=  LogicOutDataTypeMode=boolean  LogicDataType=fixdt(0, 8)  OutDataTypeStr=boolean
  Rra : Constant  Value=0.025  OutDataType=fixdt(1, 16)  OutScaling=2^0
  Subtract : Sum  Inputs=+-  OutDataType=fixdt(1, 16)  OutScaling=2^-10
  Switch : Switch  Threshold=1  OutDataType=fixdt(1, 16)  OutScaling=2^0
  Fi,r(out) : Outport  OutDataType=fixdt(1, 16)  OutScaling=2^0
  wires:
  Switch/1 -> Fi,r(out)/1
  Constant/1 -> Switch/1
  Divide/1 -> Switch/3
  Pra/1 -> Subtract/1, Relational Operator/1
  Subtract/1 -> Divide/1
  Rra/1 -> Divide/2
  Relational Operator/1 -> Switch/2
  Pmax,rv/1 -> Prv/1
  Product/1 -> Prv/2
  Rrv/1 -> Product/1
  Fo,r/1 -> Product/2
  Prv/1 -> Subtract/2, Relational Operator/2

== system simulinkCS/A1.22 ==
  Fi,r : Inport  OutDataType=fixdt(1, 16)  OutScaling=2^0
  Fo,r : Inport  Port=2  OutDataType=fixdt(1, 16)  OutScaling=2^0
  Integrator : Integrator
  Subtract : Sum  Inputs=+-  OutDataType=fixdt(1, 16)  OutScaling=2^-10
  Vrv(out) : Outport  OutDataType=fixdt(1, 16)  OutScaling=2^0
  wires:
  Integrator/1 -> Vrv(out)/1
  Fo,r/1 -> Subtract/2
  Subtract/1 -> Integrator/1
  Fi,r/1 -> Subtract/1

== system simulinkCS/A1.23 ==
  note: used A1.24
  Pmax,rv : Inport  OutDataType=fixdt(1, 16)  OutScaling=2^0
  Ppa : Inport  Port=2  OutDataType=fixdt(1, 16)  OutScaling=2^0
  Constant : Constant  Value=0  OutDataType=fixdt(1, 16)  OutScaling=2^0
  Divide : Product  Inputs=*/  OutDataType=fixdt(1, 16)  OutScaling=2^-10
  Product : Product  OutDataType=fixdt(1, 16)  OutScaling=2^0  RndMeth=Zero
  Relational Operator : RelationalOperator  Operator=<=  LogicOutDataTypeMode=boolean  LogicDataType=fixdt(0, 8)  OutDataTypeStr=boolean
  Subtract : Sum  Inputs=+-  OutDataType=fixdt(1, 16)  OutScaling=2^-10
  Switch : Switch  Threshold=1  OutDataType=fixdt(1, 16)  OutScaling=2^0
  kR,rv : Constant  Value=0.0014  OutDataType=fixdt(1, 16)  OutScaling=2^0
  Fo,r(out) : Outport  OutDataType=fixdt(1, 16)  OutScaling=2^0
  wires:
  Switch/1 -> Fo,r(out)/1
  Constant/1 -> Switch/1
  Divide/1 -> Switch/3
  Pmax,rv/1 -> Relational Operator/1, Subtract/1, Product/2
  Ppa/1 -> Subtract/2, Relational Operator/2
  Subtract/1 -> Divide/1
  Relational Operator/1 -> Switch/2
  kR,rv/1 -> Product/1
  Product/1 -> Divide/2

== system simulinkCS/A1.24 ==
  Pmax,rv : Inport  OutDataType=fixdt(1, 16)  OutScaling=2^0
  Product : Product  OutDataType=fixdt(1, 16)  OutScaling=2^0  RndMeth=Zero
  kR,rv : Constant  Value=0.0014  OutDataType=fixdt(1, 16)  OutScaling=2^0
  Rrv(out) : Outport  OutDataType=fixdt(1, 16)  OutScaling=2^0
  wires:
  Product/1 -> Rrv(out)/1
  Pmax,rv/1 -> Product/2
  kR,rv/1 -> Product/1

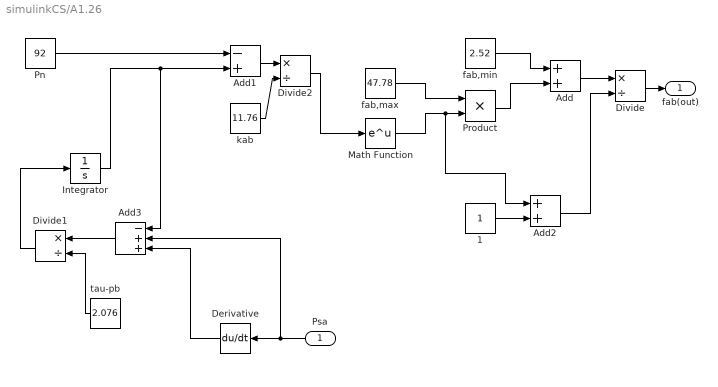
== system simulinkCS/A1.26 ==
  Psa : Inport  OutDataType=fixdt(1, 16)  OutScaling=2^0
  1 : Constant  OutDataType=fixdt(1, 16)  OutScaling=2^0
  Add : Sum  OutDataType=fixdt(1, 16)  OutScaling=2^-10
  Add1 : Sum  Inputs=-+  OutDataType=fixdt(1, 16)  OutScaling=2^-10
  Add2 : Sum  OutDataType=fixdt(1, 16)  OutScaling=2^-10
  Add3 : Sum  Inputs=-++  OutDataType=fixdt(1, 16)  OutScaling=2^-10
  Derivative : Derivative
  Divide : Product  Inputs=*/  OutDataType=fixdt(1, 16)  OutScaling=2^-10
  Divide1 : Product  Inputs=*/  OutDataType=fixdt(1, 16)  OutScaling=2^-10
  Divide2 : Product  Inputs=*/  OutDataType=fixdt(1, 16)  OutScaling=2^-10
  Integrator : Integrator
  Math Function : Math  OutDataType=fixdt(1, 16)  OutScaling=2^0  SaturateOnIntegerOverflow=on
  Pn : Constant  Value=92  OutDataType=fixdt(1, 16)  OutScaling=2^0
  Product : Product  OutDataType=fixdt(1, 16)  OutScaling=2^0  RndMeth=Zero
  fab,max : Constant  Value=47.78  OutDataType=fixdt(1, 16)  OutScaling=2^0
  fab,min : Constant  Value=2.52  OutDataType=fixdt(1, 16)  OutScaling=2^0
  kab : Constant  Value=11.76  OutDataType=fixdt(1, 16)  OutScaling=2^0
  tau-pb : Constant  Value=2.076  OutDataType=fixdt(1, 16)  OutScaling=2^0
  fab(out) : Outport  OutDataType=fixdt(1, 16)  OutScaling=2^0
  wires:
  fab,max/1 -> Product/1
  Math Function/1 -> Product/2, Add2/1
  Divide/1 -> fab(out)/1
  Add/1 -> Divide/1
  Product/1 -> Add/2
  fab,min/1 -> Add/1
  Add1/1 -> Divide2/1
  Divide2/1 -> Math Function/1
  kab/1 -> Divide2/2
  Pn/1 -> Add1/1
  1/1 -> Add2/2
  Add2/1 -> Divide/2
  Integrator/1 -> Add1/2, Add3/1
  Add3/1 -> Divide1/1
  Divide1/1 -> Integrator/1
  tau-pb/1 -> Divide1/2
  Psa/1 -> Derivative/1, Add3/2
  Derivative/1 -> Add3/3

== system simulinkCS/A1.3 ==
  Fpa : Inport  OutDataType=fixdt(1, 16)  OutScaling=2^0
  Ppv : Inport  Port=2  OutDataType=fixdt(1, 16)  OutScaling=2^0
  Cpp : Constant  Value=5.8  OutDataType=fixdt(1, 16)  OutScaling=2^0
  Divide : Product  Inputs=*/  OutDataType=fixdt(1, 16)  OutScaling=2^-10
  Divide1 : Product  Inputs=*/  OutDataType=fixdt(1, 16)  OutScaling=2^-10
  Integrator : Integrator
  Rpp : Constant  Value=0.0894  OutDataType=fixdt(1, 16)  OutScaling=2^0
  Subtract : Sum  Inputs=+-  OutDataType=fixdt(1, 16)  OutScaling=2^-10
  Subtract1 : Sum  Inputs=+-  OutDataType=fixdt(1, 16)  OutScaling=2^-10
  Ppp(out) : Outport  OutDataType=fixdt(1, 16)  OutScaling=2^0
  wires:
  Integrator/1 -> Ppp(out)/1, Subtract1/1
  Ppv/1 -> Subtract1/2
  Subtract1/1 -> Divide/1
  Fpa/1 -> Subtract/1
  Divide/1 -> Subtract/2
  Subtract/1 -> Divide1/1
  Cpp/1 -> Divide1/2
  Divide1/1 -> Integrator/1
  Rpp/1 -> Divide/2

== system simulinkCS/A1.4 ==
  Ppp : Inport  OutDataType=fixdt(1, 16)  OutScaling=2^0
  Pla : Inport  Port=2  OutDataType=fixdt(1, 16)  OutScaling=2^0
  Cpv : Constant  Value=25.37  OutDataType=fixdt(1, 16)  OutScaling=2^0
  Divide : Product  Inputs=*/  OutDataType=fixdt(1, 16)  OutScaling=2^-10
  Divide1 : Product  Inputs=*/  OutDataType=fixdt(1, 16)  OutScaling=2^-10
  Divide2 : Product  Inputs=*/  OutDataType=fixdt(1, 16)  OutScaling=2^-10
  Integrator : Integrator
  Rpp : Constant  Value=0.0894  OutDataType=fixdt(1, 16)  OutScaling=2^0
  Rpv : Constant  Value=0.0056  OutDataType=fixdt(1, 16)  OutScaling=2^0
  Subtract : Sum  Inputs=+-  OutDataType=fixdt(1, 16)  OutScaling=2^-10
  Subtract1 : Sum  Inputs=+-  OutDataType=fixdt(1, 16)  OutScaling=2^-10
  Subtract2 : Sum  Inputs=-+  OutDataType=fixdt(1, 16)  OutScaling=2^-10
  Ppv(out) : Outport  OutDataType=fixdt(1, 16)  OutScaling=2^0
  wires:
  Integrator/1 -> Subtract/2, Ppv(out)/1, Subtract2/2
  Ppp/1 -> Subtract/1
  Subtract/1 -> Divide/1
  Rpp/1 -> Divide/2
  Divide/1 -> Subtract1/1
  Subtract1/1 -> Divide1/1
  Cpv/1 -> Divide1/2
  Divide1/1 -> Integrator/1
  Pla/1 -> Subtract2/1
  Divide2/1 -> Subtract1/2
  Subtract2/1 -> Divide2/1
  Rpv/1 -> Divide2/2

== system simulinkCS/A1.5 ==
  Fo,l : Inport  OutDataType=fixdt(1, 16)  OutScaling=2^0
  Fsa : Inport  Port=2  OutDataType=fixdt(1, 16)  OutScaling=2^0
  Csa : Constant  Value=0.28  OutDataType=fixdt(1, 16)  OutScaling=2^0
  Divide : Product  Inputs=*/  OutDataType=fixdt(1, 16)  OutScaling=2^-10
  Integrator : Integrator
  Sum : Sum  Inputs=|+-  OutDataType=fixdt(1, 16)  OutScaling=2^0
  Psa(out) : Outport  OutDataType=fixdt(1, 16)  OutScaling=2^0
  wires:
  Integrator/1 -> Psa(out)/1
  Sum/1 -> Divide/1
  Divide/1 -> Integrator/1
  Csa/1 -> Divide/2
  Fsa/1 -> Sum/2
  Fo,l/1 -> Sum/1

== system simulinkCS/A1.6 ==
  Psa : Inport  OutDataType=fixdt(1, 16)  OutScaling=2^0
  Psp : Inport  Port=2  OutDataType=fixdt(1, 16)  OutScaling=2^0
  Divide : Product  Inputs=*/  OutDataType=fixdt(1, 16)  OutScaling=2^-10
  Integrator : Integrator
  Lsa : Constant  Value=0.00022  OutDataType=fixdt(1, 16)  OutScaling=2^0
  Product : Product  OutDataType=fixdt(1, 16)  OutScaling=2^0  RndMeth=Zero
  Rsa : Constant  Value=0.06  OutDataType=fixdt(1, 16)  OutScaling=2^0
  Sum : Sum  Inputs=|+--  OutDataType=fixdt(1, 16)  OutScaling=2^0
  Fsa(out) : Outport  OutDataType=fixdt(1, 16)  OutScaling=2^0
  wires:
  Integrator/1 -> Fsa(out)/1, Product/2
  Psa/1 -> Sum/1
  Psp/1 -> Sum/2
  Product/1 -> Sum/3
  Rsa/1 -> Product/1
  Sum/1 -> Divide/1
  Divide/1 -> Integrator/1
  Lsa/1 -> Divide/2

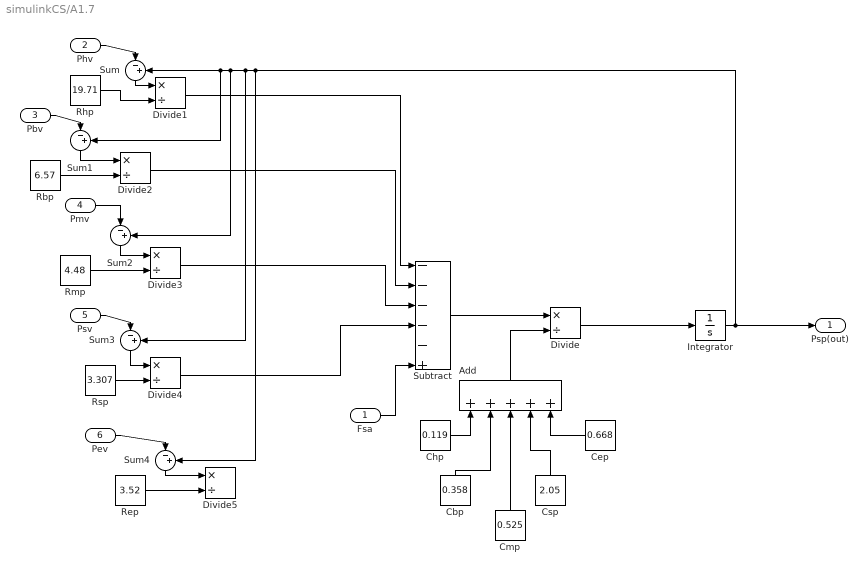
== system simulinkCS/A1.7 ==
  Fsa : Inport  OutDataType=fixdt(1, 16)  OutScaling=2^0
  Phv : Inport  Port=2  OutDataType=fixdt(1, 16)  OutScaling=2^0
  Pbv : Inport  Port=3  OutDataType=fixdt(1, 16)  OutScaling=2^0
  Pmv : Inport  Port=4  OutDataType=fixdt(1, 16)  OutScaling=2^0
  Psv : Inport  Port=5  OutDataType=fixdt(1, 16)  OutScaling=2^0
  Pev : Inport  Port=6  OutDataType=fixdt(1, 16)  OutScaling=2^0
  Add : Sum  Inputs=+++++  OutDataType=fixdt(1, 16)  OutScaling=2^-10
  Cbp : Constant  Value=0.358  OutDataType=fixdt(1, 16)  OutScaling=2^0
  Cep : Constant  Value=0.668  OutDataType=fixdt(1, 16)  OutScaling=2^0
  Chp : Constant  Value=0.119  OutDataType=fixdt(1, 16)  OutScaling=2^0
  Cmp : Constant  Value=0.525  OutDataType=fixdt(1, 16)  OutScaling=2^0
  Csp : Constant  Value=2.05  OutDataType=fixdt(1, 16)  OutScaling=2^0
  Divide{,1..5} (6 alike) : Product  Inputs=*/  OutDataType=fixdt(1, 16)  OutScaling=2^-10
  Integrator : Integrator
  Rbp : Constant  Value=6.57  OutDataType=fixdt(1, 16)  OutScaling=2^0
  Rep : Constant  Value=3.52  OutDataType=fixdt(1, 16)  OutScaling=2^0
  Rhp : Constant  Value=19.71  OutDataType=fixdt(1, 16)  OutScaling=2^0
  Rmp : Constant  Value=4.48  OutDataType=fixdt(1, 16)  OutScaling=2^0
  Rsp : Constant  Value=3.307  OutDataType=fixdt(1, 16)  OutScaling=2^0
  Subtract : Sum  Inputs=-----+  OutDataType=fixdt(1, 16)  OutScaling=2^-10
  Sum{,1..4} (5 alike) : Sum  Inputs=|-+  OutDataType=fixdt(1, 16)  OutScaling=2^0
  Psp(out) : Outport  OutDataType=fixdt(1, 16)  OutScaling=2^0
  wires:
  Integrator/1 -> Psp(out)/1, Sum/2, Sum1/2, Sum2/2, Sum3/2, Sum4/2
  Add/1 -> Divide/2
  Chp/1 -> Add/1
  Cbp/1 -> Add/2
  Cmp/1 -> Add/3
  Cep/1 -> Add/5
  Csp/1 -> Add/4
  Divide/1 -> Integrator/1
  Subtract/1 -> Divide/1
  Phv/1 -> Sum/1
  Sum/1 -> Divide1/1
  Rhp/1 -> Divide1/2
  Divide1/1 -> Subtract/1
  Pbv/1 -> Sum1/1
  Sum1/1 -> Divide2/1
  Rbp/1 -> Divide2/2
  Divide2/1 -> Subtract/2
  Fsa/1 -> Subtract/6
  Sum2/1 -> Divide3/1
  Pmv/1 -> Sum2/1
  Rmp/1 -> Divide3/2
  Divide3/1 -> Subtract/3
  Psv/1 -> Sum3/1
  Sum3/1 -> Divide4/1
  Divide4/1 -> Subtract/4
  Rsp/1 -> Divide4/2
  Sum4/1 -> Divide5/1
  Pev/1 -> Sum4/1
  Rep/1 -> Divide5/2

== system simulinkCS/A1.8 ==
  Psp : Inport  OutDataType=fixdt(1, 16)  OutScaling=2^0
  Pra : Inport  Port=2  OutDataType=fixdt(1, 16)  OutScaling=2^0
  Chv : Constant  Value=3.57  OutDataType=fixdt(1, 16)  OutScaling=2^0
  Divide : Product  Inputs=*/  OutDataType=fixdt(1, 16)  OutScaling=2^-10
  Divide1 : Product  Inputs=*/  OutDataType=fixdt(1, 16)  OutScaling=2^-10
  Divide2 : Product  Inputs=/*  OutDataType=fixdt(1, 16)  OutScaling=2^-10
  Integrator : Integrator
  Rhp : Constant  Value=19.71  OutDataType=fixdt(1, 16)  OutScaling=2^0
  Rhv : Constant  Value=0.224  OutDataType=fixdt(1, 16)  OutScaling=2^0
  Subtract : Sum  Inputs=+-  OutDataType=fixdt(1, 16)  OutScaling=2^-10
  Sum : Sum  Inputs=|+-  OutDataType=fixdt(1, 16)  OutScaling=2^0
  Sum1 : Sum  Inputs=|-+  OutDataType=fixdt(1, 16)  OutScaling=2^0
  Phv(out) : Outport  OutDataType=fixdt(1, 16)  OutScaling=2^0
  wires:
  Integrator/1 -> Phv(out)/1, Sum/2, Sum1/2
  Psp/1 -> Sum/1
  Sum/1 -> Divide1/1
  Rhp/1 -> Divide1/2
  Pra/1 -> Sum1/1
  Sum1/1 -> Divide2/2
  Rhv/1 -> Divide2/1
  Divide1/1 -> Subtract/1
  Divide2/1 -> Subtract/2
  Subtract/1 -> Divide/1
  Chv/1 -> Divide/2
  Divide/1 -> Integrator/1

== system simulinkCS/A1.9 ==
  Psp : Inport  OutDataType=fixdt(1, 16)  OutScaling=2^0
  Pra : Inport  Port=2  OutDataType=fixdt(1, 16)  OutScaling=2^0
  Cbv : Constant  Value=10.71  OutDataType=fixdt(1, 16)  OutScaling=2^0
  Divide : Product  Inputs=*/  OutDataType=fixdt(1, 16)  OutScaling=2^-10
  Divide1 : Product  Inputs=*/  OutDataType=fixdt(1, 16)  OutScaling=2^-10
  Divide2 : Product  Inputs=/*  OutDataType=fixdt(1, 16)  OutScaling=2^-10
  Integrator : Integrator
  Rbp : Constant  Value=6.57  OutDataType=fixdt(1, 16)  OutScaling=2^0
  Rbv : Constant  Value=0.075  OutDataType=fixdt(1, 16)  OutScaling=2^0
  Subtract : Sum  Inputs=+-  OutDataType=fixdt(1, 16)  OutScaling=2^-10
  Sum : Sum  Inputs=|+-  OutDataType=fixdt(1, 16)  OutScaling=2^0
  Sum1 : Sum  Inputs=|-+  OutDataType=fixdt(1, 16)  OutScaling=2^0
  Pbv(out) : Outport  OutDataType=fixdt(1, 16)  OutScaling=2^0
  wires:
  Integrator/1 -> Pbv(out)/1, Sum/2, Sum1/2
  Psp/1 -> Sum/1
  Sum/1 -> Divide1/1
  Rbp/1 -> Divide1/2
  Pra/1 -> Sum1/1
  Sum1/1 -> Divide2/2
  Rbv/1 -> Divide2/1
  Divide1/1 -> Subtract/1
  Divide2/1 -> Subtract/2
  Subtract/1 -> Divide/1
  Cbv/1 -> Divide/2
  Divide/1 -> Integrator/1

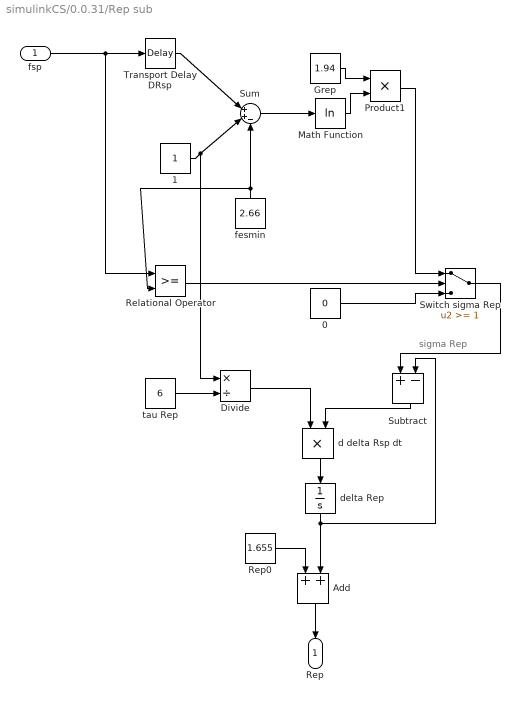
== system simulinkCS/0.0.31/Rep sub ==
  note: sigma Rep
  fsp : Inport  OutDataType=sfix(16)  OutScaling=2^0
  0 : Constant  Value=0  OutDataType=sfix(16)  OutScaling=2^0
  1 : Constant  OutDataType=sfix(16)  OutScaling=2^0
  Add : Sum  OutDataType=sfix(16)  OutScaling=2^-10
  Divide : Product  Inputs=*/  OutDataType=sfix(16)  OutScaling=2^-10
  Grep : Constant  Value=1.94  OutDataType=sfix(16)  OutScaling=2^0
  Math Function : Math  Operator=log  OutDataType=sfix(16)  OutScaling=2^0  SaturateOnIntegerOverflow=on
  Product1 : Product  OutDataType=sfix(16)  OutScaling=2^0  RndMeth=Zero
  Relational Operator : RelationalOperator  LogicOutDataTypeMode=boolean  OutDataTypeStr=boolean
  Rep0 : Constant  Value=1.655  OutDataType=sfix(16)  OutScaling=2^0
  Subtract : Sum  Inputs=+-  OutDataType=sfix(16)  OutScaling=2^-10
  Sum : Sum  Inputs=|++-  OutDataType=sfix(16)  OutScaling=2^0
  Switch sigma Rep : Switch  Threshold=1
  Transport Delay DRsp : TransportDelay  DelayTime=2
  "d delta Rsp dt  " : Product  OutDataType=sfix(16)  OutScaling=2^0  RndMeth=Zero
  delta Rep : Integrator
  fesmin : Constant  Value=2.66  OutDataType=sfix(16)  OutScaling=2^0
  tau Rep : Constant  Value=6  OutDataType=sfix(16)  OutScaling=2^0
  Rep : Outport  OutDataType=sfix(16)  OutScaling=2^0
  wires:
  fsp/1 -> Transport Delay DRsp/1, Relational Operator/1
  Grep/1 -> Product1/1
  1/1 -> Sum/2, Divide/1
  fesmin/1 -> Sum/3, Relational Operator/2
  Transport Delay DRsp/1 -> Sum/1
  Sum/1 -> Math Function/1
  Math Function/1 -> Product1/2
  Product1/1 -> Switch sigma Rep/1
  Relational Operator/1 -> Switch sigma Rep/2
  0/1 -> Switch sigma Rep/3
  Switch sigma Rep/1 -> Subtract/1
  tau Rep/1 -> Divide/2
  delta Rep/1 -> Subtract/2, Add/2
  Subtract/1 -> "d delta Rsp dt  "/2
  Divide/1 -> "d delta Rsp dt  "/1
  "d delta Rsp dt  "/1 -> delta Rep/1
  Rep0/1 -> Add/1
  Add/1 -> Rep/1
